simulink model "flexpwm_ctu_adc_block"  (Simulink 8.1)
settings: Solver=FixedStepDiscrete  StartTime=0.0  StopTime=10.0  FixedStep=0.2  RelTol=1e-3
undefined symbols (not defined in the file or in its folder): A14, A15, AN1, AN12, AN2, AN3, AN4, B, B13, B7, D, L3, M3, P11, P3, PB10, PB14, PB15, PC10, PC14, PC2, PD4, PD6, PD8, PE6, R10, R11, R6, R8, U5
libraries: rappid_564xl_ec_toolbox x13
settings Model: Creator=evarshavskaya  LastModifiedBy=evarshavskaya
settings DataIOCC: ExternalInput=off  InitialState=off  SaveOutput=off  SignalLogging=off  SaveTime=off
settings OptimizationCC: InlineParams=on  OptimizeModelRefInitCode=on  LifeSpan=1
settings DebuggingCC: InheritedTsInSrcMsg=none  SingleTaskRateTransMsg=error  UnconnectedInputMsg=error  UnconnectedOutputMsg=error  UnconnectedLineMsg=error  UnknownTsInhSupMsg=error
settings HardwareCC: ProdLargestAtomicInteger=Long  ProdLargestAtomicFloat=Double  ProdIntDivRoundTo=Zero  ProdEndianess=BigEndian  ProdHWDeviceType=Freescale->32-bit PowerPC
settings RTWCC: SystemTargetFile=rappid564xl.tlc  MakeCommand=rappid_564xl_make_rtw  TemplateMakefile=rappid_564xl_default_tmf  PostCodeGenCommand=rappid_analyzegencode(buildInfo)  Description=RAppID Toolbox MPC564xL Code Generation Target (rappid)  ProcessScript=rappid564xl_make_rtw_hook
settings CodeAppCC: IgnoreCustomStorageClasses=off  CustomSymbolStrType=$N$R$M  InternalIdentifier=Classic
settings STFCustomTargetCC: CodeReplacementLibrary=ANSI_C  ModelReferenceCompliant=off  CombineOutputUpdateFcns=on  SuppressErrorStatus=on  ERTCustomFileBanners=on  SupportContinuousTime=off  SupportNonInlinedSFcns=off  MATLABClassNameForMDSCustomization=Simulink.SoftwareTarget.ERTCustomization  GRTInterface=off  SystemTargetFile=rappid564xl.tlc
settings ERTTargetCC: CodeReplacementLibrary=ANSI_C  MultiwordLength=2048  ModelReferenceCompliant=off  ParMdlRefBuildCompliant=off  CompOptLevelCompliant=off  ConcurrentExecutionCompliant=off  SuppressErrorStatus=on  ERTFirstTimeCompliant=off  ModelStepFunctionPrototypeControlCompliant=off  CPPClassGenCompliant=off  ExtModeMexFile=noextcomm  InlinedParameterPlacement=NonHierarchical  ERTCustomFileTemplate=example_file_process.tlc  ConvertIfToSwitch=off  SuppressUnreachableDefaultCases=off

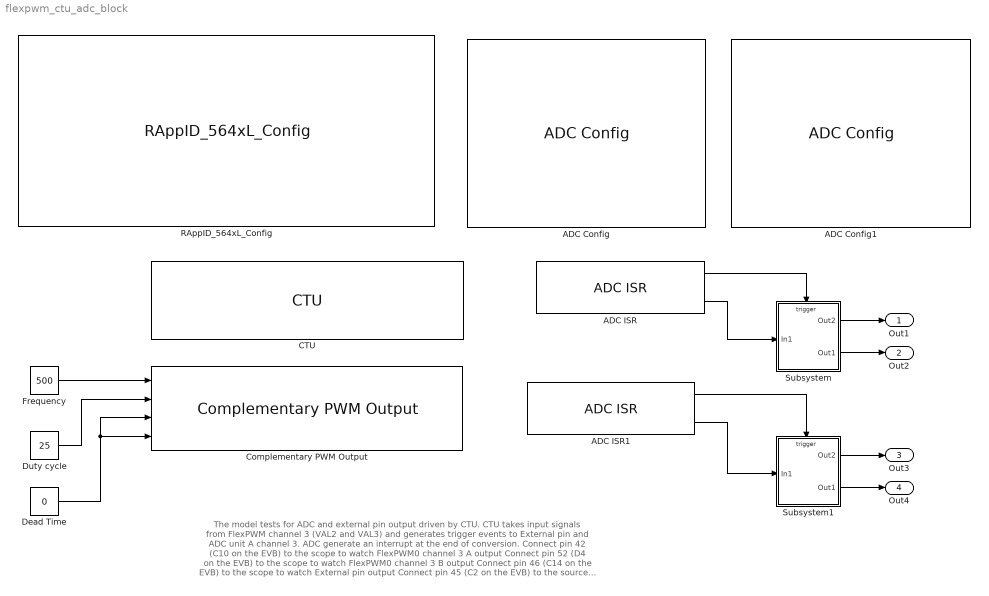
== system flexpwm_ctu_adc_block ==
  note: The model tests for ADC and external pin output driven by CTU.
      |
      | CTU takes input signals from FlexPWM channel 3 (VAL2 and VAL3) and generates trigger events
      | to External pin and ADC unit A channel 3. ADC generate an interrupt at the end of conversion.
      |
      | Connect pin 42 (C10 on the EVB) to the scope to watch FlexPWM0 channel 3 A output
      | Connect pin 52 (D4 on the EVB) to the scope to watch FlexPWM0 channel 3 B output
      | Connect pin 46 (C14 on the EVB) to the scope to watch External pin output
      | Connect pin 45 (C2 on the EVB) to the source of the signal (pin C14 as example) to provide data to the ADC0 Channel 3.
  ADC Config : rappid_564xl_ec_toolbox/MPC564xL/Motor Control Blocks/ADC Config  adc_unit=0  adc_ctu=on  adc_owr=on  adc_wls=Left  adc_clk=on  adc_ack=on  adc_ctr0_inp=off  adc_ctr0_shft=10 - Avin = 0  adc_ctr0_cmp=01  adc_ctr0_samp=4  adc_ctr1_inp=off  adc_ctr1_cmp=01  adc_ctr1_samp=1  adc_ctr1_tsens=PTAT  adc_pscr_preval=V0  adc_pscr_preconv=off
  ADC Config1 : rappid_564xl_ec_toolbox/MPC564xL/Motor Control Blocks/ADC Config  adc_unit=1  adc_ctu=on  adc_owr=on  adc_wls=Left  adc_clk=on  adc_ack=on  adc_ctr0_inp=off  adc_ctr0_shft=10 - Avin = 0  adc_ctr0_cmp=01  adc_ctr0_samp=4  adc_ctr1_inp=off  adc_ctr1_cmp=01  adc_ctr1_samp=1  adc_ctr1_tsens=PTAT  adc_pscr_preval=V0  adc_pscr_preconv=off
  ADC ISR : rappid_564xl_ec_toolbox/MPC564xL/Motor Control Blocks/ADC ISR  adc_unit=0  adc_isr_pri=15  adc_isr_ech=off  adc_isr_eoc=off  adc_isr_jech=off  adc_isr_jeoc=off  adc_isr_eoctu=on
  ADC ISR1 : rappid_564xl_ec_toolbox/MPC564xL/Motor Control Blocks/ADC ISR  adc_unit=1  adc_isr_pri=15  adc_isr_ech=off  adc_isr_eoc=off  adc_isr_jech=off  adc_isr_jeoc=off  adc_isr_eoctu=on
  CTU : rappid_564xl_ec_toolbox/MPC564xL/Motor Control Blocks/CTU  ModeEdit=Triggered  Mode=0  MRSedit=PWM reload Rising edge  MRS=0  MaxDelay=1000  ExtTgrPin_0="46  : PC14 : [ 103 ] : [ E15 ]"  ExtInPin_0=None  extTgrPcr=46  extInPcr=255  InputSelection=65536  PWM_REL=Disabled  PWM_ODD_0=Disabled  PWM_ODD_1=Disabled  PWM_ODD_2=Disabled  PWM_ODD_3=Disabled  PWM_EVEN_0=Disabled  PWM_EVEN_1=Disabled  PWM_EVEN_2=Disabled  PWM_EVEN_3=Rising  RPWM_0=Disabled  RPWM_1=Disabled  RPWM_2=Disabled  RPWM_3=Disabled  eTimer_0=Disabled  eTimer_1=Disabled  External=Disabled  TriggerOutput_1=24929  TriggerOutput_2=0  ADC_CmdIndex_1=512  ADC_CmdIndex_2=0  ADC_Cmd_1=16387  ADC_Cmd_2=4  ADC_Cmd_3=16417  ADC_Cmd_4=34  ADC_Cmd_5=16384  ADC_Cmd_6=0  ADC_Cmd_7=0  ADC_Cmd_8=0  ADC_Cmd_9=0  ADC_Cmd_10=0  ADC_Cmd_11=0  ADC_Cmd_12=0  ADC_Cmd_13=0  ADC_Cmd_14=0  ADC_Cmd_15=0  ADC_Cmd_16=0  ADC_Cmd_17=0  ADC_Cmd_18=0  ADC_Cmd_19=0  ADC_Cmd_20=0  ADC_Cmd_21=0  ADC_Cmd_22=0  ADC_Cmd_23=0  ADC_Cmd_24=0  T0_E=on  T0_ETE=on  T0_T0E=off  T0_T1E=off  T0_T2E=off  T0_ADCE=on  T0_Delay=300  T1_E=on  T1_ETE=on  T1_T0E=off  T1_T1E=off  T1_T2E=off  T1_ADCE=on  T1_Delay=500  T2_E=off  T2_ETE=off  T2_T0E=off  T2_T1E=off  T2_T2E=off  T2_ADCE=off  T2_Delay=0  T3_E=off  T3_ETE=off  T3_T0E=off  T3_T1E=off  T3_T2E=off  T3_ADCE=off  T3_Delay=0  T4_E=off  T4_ETE=off  T4_T0E=off  T4_T1E=off  T4_T2E=off  T4_ADCE=off  T4_Delay=0  T5_E=off  T5_ETE=off  T5_T0E=off  T5_T1E=off  T5_T2E=off  T5_ADCE=off  T5_Delay=0  T6_E=off  T6_ETE=off  T6_T0E=off  T6_T1E=off  T6_T2E=off  T6_ADCE=off  T6_Delay=0  T7_E=off  T7_ETE=off  T7_T0E=off  T7_T1E=off  T7_T2E=off  T7_ADCE=off  T7_Delay=0  T_delay=0  ADC_Cmd=0  T0_ADC_num=2  T0_ADC_nlist=1...2  T1_ADC_num=2  T1_ADC_nlist=3...4  T2_ADC_num=0  T2_ADC_nlist=no commands  T3_ADC_num=0  T3_ADC_nlist=no commands  T4_ADC_num=0  T4_ADC_nlist=no commands  T5_ADC_num=0  T5_ADC_nlist=no commands  T6_ADC_num=0  T6_ADC_nlist=no commands  T7_ADC_num=0  T7_ADC_nlist=no commands  ADC_CMS_1=Single-conversion mode: ADC unit A  ADC_CIR_1=Disabled  ADC_FIFO_1=0  ADC_CHA_1=3  ADC_CHB_1=0  ADC_CMS_2=Single-conversion mode: ADC unit A  ADC_CIR_2=Disabled  ADC_FIFO_2=0  ADC_CHA_2=4  ADC_CHB_2=0  ADC_CMS_3=Single-conversion mode: ADC unit B  ADC_CIR_3=Disabled  ADC_FIFO_3=0  ADC_CHA_3=0  ADC_CHB_3=1  ADC_CMS_4=Single-conversion mode: ADC unit B  ADC_CIR_4=Disabled  ADC_FIFO_4=0  ADC_CHA_4=0  ADC_CHB_4=2  ADC_CMS_5=Single-conversion mode: ADC unit A  ADC_CIR_5=Disabled  ADC_FIFO_5=0  ADC_CHA_5=0  ADC_CHB_5=0  ADC_CMS_6=Single-conversion mode: ADC unit A  ADC_CIR_6=Disabled  ADC_FIFO_6=0  ADC_CHA_6=0  ADC_CHB_6=0  ADC_CMS_7=Single-conversion mode: ADC unit A  ADC_CIR_7=Disabled  ADC_FIFO_7=0  ADC_CHA_7=0  ADC_CHB_7=0  ADC_CMS_8=Single-conversion mode: ADC unit A  ADC_CIR_8=Disabled  ADC_FIFO_8=0  ADC_CHA_8=0  ADC_CHB_8=0  ADC_CMS_9=Single-conversion mode: ADC unit A  ADC_CIR_9=Disabled  ADC_FIFO_9=0  ADC_CHA_9=0  ADC_CHB_9=0  ADC_CMS_10=Single-conversion mode: ADC unit A  ADC_CIR_10=Disabled  ADC_FIFO_10=0  ADC_CHA_10=0  ADC_CHB_10=0  ADC_CMS_11=Single-conversion mode: ADC unit A  ADC_CIR_11=Disabled  ADC_FIFO_11=0  ADC_CHA_11=0  ADC_CHB_11=0  ADC_CMS_12=Single-conversion mode: ADC unit A  ADC_CIR_12=Disabled  ADC_FIFO_12=0  ADC_CHA_12=0  ADC_CHB_12=0  ADC_CMS_13=Single-conversion mode: ADC unit A  ADC_CIR_13=Disabled  ADC_FIFO_13=0  ADC_CHA_13=0  ADC_CHB_13=0  ADC_CMS_14=Single-conversion mode: ADC unit A  ADC_CIR_14=Disabled  ADC_FIFO_14=0  ADC_CHA_14=0  ADC_CHB_14=0  ADC_CMS_15=Single-conversion mode: ADC unit A  ADC_CIR_15=Disabled  ADC_FIFO_15=0  ADC_CHA_15=0  ADC_CHB_15=0  ADC_CMS_16=Single-conversion mode: ADC unit A  ADC_CIR_16=Disabled  ADC_FIFO_16=0  ADC_CHA_16=0  ADC_CHB_16=0  ADC_CMS_17=Single-conversion mode: ADC unit A  ADC_CIR_17=Disabled  ADC_FIFO_17=0  ADC_CHA_17=0  ADC_CHB_17=0  ADC_CMS_18=Single-conversion mode: ADC unit A  ADC_CIR_18=Disabled  ADC_FIFO_18=0  ADC_CHA_18=0  ADC_CHB_18=0  ADC_CMS_19=Single-conversion mode: ADC unit A  ADC_CIR_19=Disabled  ADC_FIFO_19=0  ADC_CHA_19=0  ADC_CHB_19=0  ADC_CMS_20=Single-conversion mode: ADC unit A  ADC_CIR_20=Disabled  ADC_FIFO_20=0  ADC_CHA_20=0  ADC_CHB_20=0  ADC_CMS_21=Single-conversion mode: ADC unit A  ADC_CIR_21=Disabled  ADC_FIFO_21=0  ADC_CHA_21=0  ADC_CHB_21=0  ADC_CMS_22=Single-conversion mode: ADC unit A  ADC_CIR_22=Disabled  ADC_FIFO_22=0  ADC_CHA_22=0  ADC_CHB_22=0  ADC_CMS_23=Single-conversion mode: ADC unit A  ADC_CIR_23=Disabled  ADC_FIFO_23=0  ADC_CHA_23=0  ADC_CHB_23=0  ADC_CMS_24=Single-conversion mode: ADC unit A  ADC_CIR_24=Disabled  ADC_FIFO_24=0  ADC_CHA_24=0  ADC_CHB_24=0  dst=|  T0_cmdNum=0  T0_ADC_CMS_1=Single-conversion mode: ADC unit A  T0_ADC_CIR_1=Disabled  T0_ADC_FIFO_1=0  T0_ADC_CHA_1=3  T0_ADC_CHB_1=0  T0_ADC_CMS_2=Single-conversion mode: ADC unit A  T0_ADC_CIR_2=Disabled  T0_ADC_FIFO_2=0  T0_ADC_CHA_2=0  T0_ADC_CHB_2=0  T0_ADC_CMS_3=Single-conversion mode: ADC unit A  T0_ADC_CIR_3=Disabled  T0_ADC_FIFO_3=0  T0_ADC_CHA_3=0  T0_ADC_CHB_3=0  T1_cmdNum=0  T1_ADC_CMS_1=Single-conversion mode: ADC unit A  T1_ADC_CIR_1=Disabled  T1_ADC_FIFO_1=0  T1_ADC_CHA_1=3  T1_ADC_CHB_1=0  T1_ADC_CMS_2=Single-conversion mode: ADC unit A  T1_ADC_CIR_2=Disabled  T1_ADC_FIFO_2=0  T1_ADC_CHA_2=0  T1_ADC_CHB_2=0  T1_ADC_CMS_3=Single-conversion mode: ADC unit A  T1_ADC_CIR_3=Disabled  T1_ADC_FIFO_3=0  T1_ADC_CHA_3=0  T1_ADC_CHB_3=0  ver=2
      | Triggered mode
      |       Input selection: 00000000 00000001 00000000 00000000
      | Trigger Output 0-3: 00000000 00000000 01100001 01100001
      | Trigger Output 4-7: 00000000 00000000 00000000 00000000
      | ADC command list size: 4
  Complementary PWM Output : rappid_564xl_ec_toolbox/MPC564xL/Motor Control Blocks/Complementary PWM Output  pwmModule=0  pwmMod=0  SubModule=3  subMod=3  InitFreq=500  resolution=1 %  resValue=1  InitDuty=25  pwm45=off  pwm45en=0  InitDutyB=0  DeadTime=0  dt=IPBus clock cycles  deadtime_mks=0  debugSw=off  debug_mode=0  pin_A0=None  pin_B0=None  pin_A1=None  pin_B1=None  pin_A2=None  pin_B2=None  pin_A3="42  : PC10 : [ 111 ] : [ A15 ]"  pin_B3="52  : PD4  : [ 129 ] : [ B7 ]"  pin1_A0=None  pin1_B0=None  pin1_A1=None  pin1_B1=None  pin1_A2=None  pin1_B2=None  pin1_A3=None  pin1_B3=None  pcrNumA=42  pcrNumB=52  polA=off  polB=off  octrl=0  syncFrom0=off  masterSync=0  outVal0=off  outVal1=off  outVal2=on  outVal3=on  outVal4=on  outVal5=on  outTrig=12
  Dead Time : Constant  Value=0  OutDataTypeStr=uint32
  Duty cycle : Constant  Value=25  OutDataTypeStr=uint32
  Frequency : Constant  Value=500  OutDataTypeStr=uint32
  RAppID_564xL_Config : rappid_564xl_ec_toolbox/MPC564xL/RAppID_564xL_Config  SystemClock=120  XTAL=40  MC_clock_60=12  MC_clock_80=16  MC_clock_120=10  SWG_clock_60=20  SWG_clock_80=13.334  SWG_clock_120=20  Compiler=CodeWarrior  MemTarget=RAM  Part=MPC5643L  Package=144 LQFP  global_int_priority=10  base_tick_priority=14  sys_task_supress=off  exception_handlers=off  stored_mdl_name=flexpwm_ctu_adc_block  freemaster_interface=Oops  freemaster_rx_pin="LINFlex_0 Rx Pin 116 : \"PB[3]\""  freemaster_tx_pin="LINFlex_0 Tx Pin 114 : \"PB[2]\""  freemaster_interface_1=None  freemaster_enable=off  freemaster_rate=57600  freemaster_tx0_pin=18 : B[2] : 114 : A14  freemaster_rx0_pin=19 : B[3] : 116 : B13  freemaster_tx1_pin=57 : D[9] : 26 : L3  freemaster_rx1_pin=29 : B[13] : 60 : R10  freemaster_can_channel=1CH  freemater_can_speed=500K  freemaster_can_msgig=0x7AA  ccp_interface=None  ccp_enable=off  ccp_can_channel=CH1 (MB 0 - 1)  ccp_can_speed=500K  ccp_can_cro_id=256  ccp_can_dto_id=257  ccp_dev_id=RappID  ccp_dev_addr=0  ccp_odt=3  ccp_daq=3  pil_enable=off  pil_bam=on  comport=1  pil_rate=57600  bam_password_def=on  bam_password=0xFEEDFACECAFEBEEF  bam_sa_cs=off  bam_start_address=0x0  bam_code_size=0x7000  cons_dspi=on  cons_can=on  cons_adc=on  cons_pwm=on  cons_ctu=on  cons_swg=on  cons_eTimer=on  cons_fm=on
  Subsystem : Subsystem
      settings: RTWSystemCode=Nonreusable function
  Subsystem1 : Subsystem
      settings: RTWSystemCode=Nonreusable function
  Out1 : Outport
  Out2 : Outport  Port=2
  Out3 : Outport  Port=3
  Out4 : Outport  Port=4
  wires:
  Frequency/1 -> Complementary PWM Output/1
  Duty cycle/1 -> Complementary PWM Output/2
  Dead Time/1 -> Complementary PWM Output/3, Complementary PWM Output/4
  ADC ISR/1 -> Subsystem/Trigger
  Subsystem/1(Out2) -> Out1/1
  ADC ISR/2 -> Subsystem/1(In1)
  Subsystem/2(Out1) -> Out2/1
  ADC ISR1/1 -> Subsystem1/Trigger
  Subsystem1/1(Out2) -> Out3/1
  ADC ISR1/2 -> Subsystem1/1(In1)
  Subsystem1/2(Out1) -> Out4/1

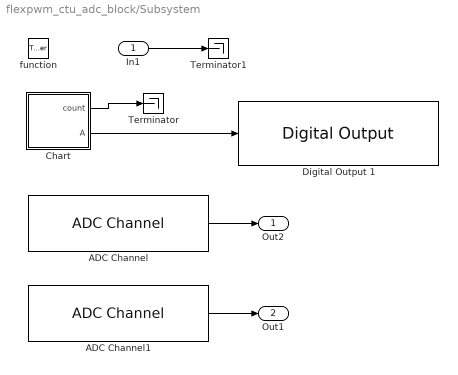
== system flexpwm_ctu_adc_block/Subsystem ==
  In1 : Inport
  function : TriggerPort  TriggerType=function-call
  ADC Channel : rappid_564xl_ec_toolbox/MPC564xL/Motor Control Blocks/ADC Channel  adc_unit=0  adc_chan0=older  adc_chan0_v2=34 : PC2 : [45] : [U5] : AN3  adc_chan1=older  adc_chan1_v2=26 : PB10 : [53] : [R8] : AN12  simulate=off  interrupt=on  adc_mode=Normal  adc_presample=off
  ADC Channel1 : rappid_564xl_ec_toolbox/MPC564xL/Motor Control Blocks/ADC Channel  adc_unit=0  adc_chan0=older  adc_chan0_v2=70 : PE6 : [46] : [R6] : AN4  adc_chan1=older  adc_chan1_v2=26 : PB10 : [53] : [R8] : AN12  simulate=off  interrupt=on  adc_mode=Normal  adc_presample=off
  Chart : Stateflow chart  TreatAsAtomicUnit=on
  Digital Output 1 : rappid_564xl_ec_toolbox/MPC564xL/General Purpose Blocks/Digital Output   gpio_outputs="54  : PD6  : [ 34 ] : [ P3 ]"  pinNum=[ 34 ]  pcrNum=54
  Terminator : Terminator
  Terminator1 : Terminator
  Out2 : Outport
  Out1 : Outport  Port=2
  wires:
  ADC Channel/1 -> Out2/1
  Chart/2(A) -> Digital Output 1/1
  Chart/1(count) -> Terminator/1
  In1/1 -> Terminator1/1
  ADC Channel1/1 -> Out1/1

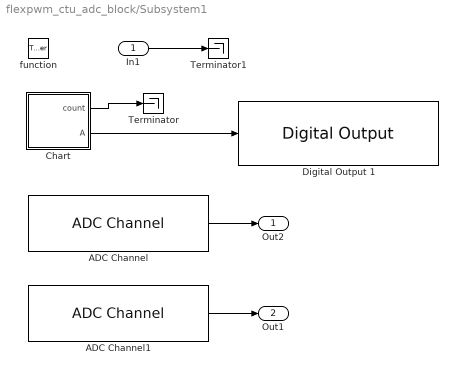
== system flexpwm_ctu_adc_block/Subsystem1 ==
  In1 : Inport
  function : TriggerPort  TriggerType=function-call
  ADC Channel : rappid_564xl_ec_toolbox/MPC564xL/Motor Control Blocks/ADC Channel  adc_unit=1  adc_chan0=older  adc_chan0_v2=34 : PC2 : [45] : [U5] : AN3  adc_chan1=older  adc_chan1_v2=30 : PB14 : [64] : [P11] : AN1  simulate=off  interrupt=on  adc_mode=Normal  adc_presample=off
  ADC Channel1 : rappid_564xl_ec_toolbox/MPC564xL/Motor Control Blocks/ADC Channel  adc_unit=1  adc_chan0=older  adc_chan0_v2=70 : PE6 : [46] : [R6] : AN4  adc_chan1=older  adc_chan1_v2=31 : PB15 : [62] : [R11] : AN2  simulate=off  interrupt=on  adc_mode=Normal  adc_presample=off
  Chart : Stateflow chart  TreatAsAtomicUnit=on
  Digital Output 1 : rappid_564xl_ec_toolbox/MPC564xL/General Purpose Blocks/Digital Output   gpio_outputs="56  : PD8  : [ 32 ] : [ M3 ]"  pinNum=[ 32 ]  pcrNum=56
  Terminator : Terminator
  Terminator1 : Terminator
  Out2 : Outport
  Out1 : Outport  Port=2
  wires:
  ADC Channel/1 -> Out2/1
  Chart/2(A) -> Digital Output 1/1
  Chart/1(count) -> Terminator/1
  In1/1 -> Terminator1/1
  ADC Channel1/1 -> Out1/1

== stateflow chart Subsystem1/Chart ==
  state A
  state A1
  (default) -> A : {count =0;}
  A -> A1
  A1 -> A : { count = count + 1;}
  data: count output double; A output boolean

== stateflow chart Subsystem/Chart ==
  state A
  state A1
  (default) -> A : {count =0;}
  A -> A1
  A1 -> A : { count = count + 1;}
  data: count output double; A output boolean
